simulink model "Vehicle_long_dyn_LinearizedModel"  (R2020b)
settings: Solver=VariableStepAuto  StartTime=0.0  StopTime=200  RelTol=1e-3
values from neighbouring files (symbols this model uses):
  A = 2.24    [Vehicle_longitudinal_dynamics.m]
  Cd = 0.3    [Vehicle_longitudinal_dynamics.m]
  g = 9.81    [Vehicle_longitudinal_dynamics.m]
  m = 1084    [Vehicle_longitudinal_dynamics.m]
  rho = 1.2    [Vehicle_longitudinal_dynamics.m]
  V0 = 22    [Vehicle_longitudinal_dynamics.m]
  Vw_0 = 1.2    [Vehicle_longitudinal_dynamics.m]
settings Model: Creator=ChOm1  LastModifiedBy=ChOm1

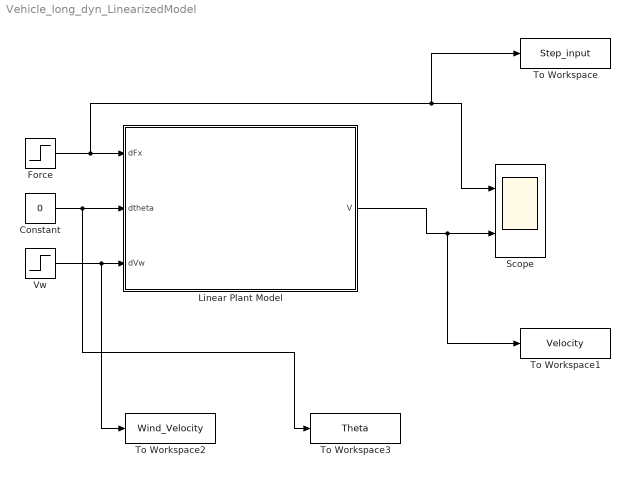
== system Vehicle_long_dyn_LinearizedModel ==
  Constant : Constant  Value=0
  Force : Step  SampleTime=0
  Linear Plant Model : Subsystem
  Scope : Scope  NumInputPorts=2
  To Workspace : ToWorkspace  VariableName=Step_input  SaveFormat=Timeseries  SampleTime=-1
  To Workspace1 : ToWorkspace  VariableName=Velocity  SaveFormat=Timeseries  SampleTime=-1
  To Workspace2 : ToWorkspace  VariableName=Wind_Velocity  SaveFormat=Timeseries  SampleTime=-1
  To Workspace3 : ToWorkspace  VariableName=Theta  SaveFormat=Timeseries  SampleTime=-1
  Vw : Step  SampleTime=0
  wires:
  Force/1 -> To Workspace/1, Scope/1, Linear Plant Model/1(dFx)
  Constant/1 -> To Workspace3/1, Linear Plant Model/2(dtheta)
  Vw/1 -> To Workspace2/1, Linear Plant Model/3(dVw)
  Linear Plant Model/1(V) -> To Workspace1/1, Scope/2

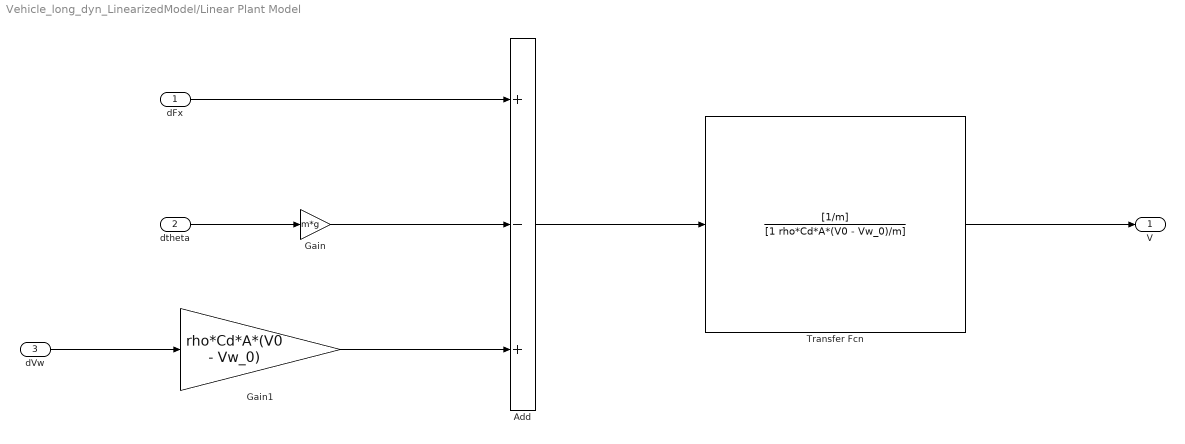
== system Vehicle_long_dyn_LinearizedModel/Linear Plant Model ==
  dFx : Inport
  dtheta : Inport  Port=2
  dVw : Inport  Port=3
  Add : Sum  Inputs=+-+
  Gain : Gain  Gain=m*g
  Gain1 : Gain  Gain=rho*Cd*A*(V0 - Vw_0)
  Transfer Fcn : TransferFcn  Numerator=[1/m]  Denominator=[1 rho*Cd*A*(V0 - Vw_0)/m]
  V : Outport
  wires:
  dtheta/1 -> Gain/1
  Gain/1 -> Add/2
  dFx/1 -> Add/1
  Gain1/1 -> Add/3
  dVw/1 -> Gain1/1
  Add/1 -> Transfer Fcn/1
  Transfer Fcn/1 -> V/1
